simulink model "rtwdemo_slcustcode"  (Simulink 7.6)
settings: Solver=FixedStepDiscrete  StartTime=0.0  StopTime=48  FixedStep=1  RelTol=1e-3
libraries: rtwdemowidgets x3
Description:
  | Integrating Legacy Code Using Custom Code Blocks
settings Model: Creator=The MathWorks Inc.  ParamWorkspaceSource=ReferencedWorkspace  CovMetricSettings=d  ExtModeTrigMode=oneshot  ExtModeArmWhenConnect=off  ExtModeAutoUpdateStatusClock=off
settings MATStruct: SampleTime=1  Offset=0  Priority=[20.0]
settings DataIOCC: LimitDataPoints=off  SaveFormat=StructureWithTime  SaveOutput=off  SaveTime=off  SignalLoggingName=sigsOut
settings OptimizationCC: InlineParams=on  InlineInvariantSignals=on  StateBitsets=on  DataBitsets=on  UseTempVars=on  EfficientFloat2IntCast=on  EfficientMapNaN2IntZero=off
settings DebuggingCC: CheckExecutionContextPreStartOutputMsg=on  CheckExecutionContextRuntimeOutputMsg=on  SolverPrmCheckMsg=none  IntegerOverflowMsg=none  StrictBusMsg=ErrorOnBusTreatedAsVector
settings HardwareCC: ProdIntDivRoundTo=Zero  ProdEndianess=LittleEndian  ProdHWDeviceType=Generic->32-bit Embedded Processor  TargetHWDeviceType=Generic->32-bit Embedded Processor
settings ModelReferenceCC: UpdateModelReferenceTargets=IfOutOfDate
settings RTWCC: TLCOptions=-p0 -aWarnNonSaturatedBlocks=0  GenerateReport=on  RTWVerbose=off  ProcessScript=grt_make_rtw_hook  LaunchReport=on
settings RTWCC: CustomSourceCode=|
  | /* Declared from Configration Parameters RTW Custom Code Page (Source file) */
  | int_T GLOBAL_INT2 = -1;
settings RTWCC: CustomInitializer=|
  | /* Declared from Configuration Parameters RTW Custom Code Page (Initialize function) */
  | GLOBAL_INT2 = 1;
settings CodeAppCC: ForceParamTrailComments=on
settings GRTTargetCC: TargetFcnLib=ansi_tfl_tmw.mat

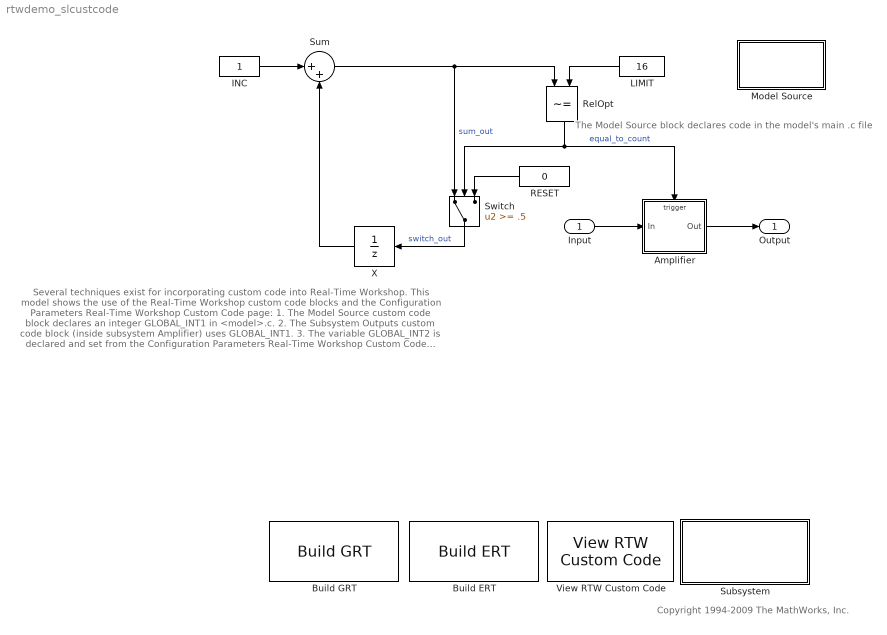
== system rtwdemo_slcustcode ==
  note: Several techniques exist for incorporating custom code into Real-Time Workshop.  This model
      | shows the use of the Real-Time Workshop custom code blocks and the Configuration Parameters
      | Real-Time Workshop Custom Code page:
      |
      | 1. The Model Source custom code block declares an integer GLOBAL_INT1 in <model>.c.
      | 2. The Subsystem Outputs custom code block (inside subsystem Amplifier) uses GLOBAL_INT1.
      | 3. The variable GLOBAL_INT2 is declared and set from the Configuration Parameters Real-Time
      |     Workshop Custom Code page, from the "Source file" and "Initialize function," respectively.
      |
      | Some overlap exists between custom code blocks and custom code specified using configuration
      | parameters, but custom code blocks provide much finer granularity of code placement, and have
      | the advantage of being graphical.
  note: The Model Source block
      | declares code in the
      | model's main .c file
  note: Copyright 1994-2009 The MathWorks, Inc.
  Input : Inport  OutDataTypeStr=int32  PortDimensions=1  SampleTime=1
  Amplifier : Subsystem  TreatAsAtomicUnit=on
  Build ERT : rtwdemowidgets/Build ERT  SystemSampleTime=-1  attrib_overrides={'IncludeMdlTerminateFcn'}
  Build GRT : rtwdemowidgets/Build GRT  SystemSampleTime=-1  attrib_overrides={}
  INC : Constant
  LIMIT : Constant  Value=16
  Model Source : Subsystem
      settings: CopyFcn=cccopyfcn(gcb)  OpenFcn=ccopenfcn('Model Source')
      mask Type: Model Source
      mask Description: Add code to the model .c file
      mask Help: This source file block contains text fields to insert custom user code at the top and bottom of model.c file.
      mask Display: disp('Model\nSource');
  RESET : Constant  Value=0
  RelOpt : RelationalOperator  Operator=~=  InputSameDT=on
  Subsystem : Subsystem
      settings: OpenFcn=custcode
      mask Display:
      | disp(['View Custom\nCode ',...
      | 	  'Library\n(double-click)'])
  Sum : Sum  Inputs=|++  InputSameDT=on  OutDataTypeStr=Inherit: Same as first input
  Switch : Switch  Threshold=.5  SaturateOnIntegerOverflow=on  InputSameDT=on
  View RTW Custom Code : rtwdemowidgets/View RTW Custom Code  SystemSampleTime=-1
  X : UnitDelay  StateIdentifier=X
  Output : Outport
  wires:
  INC/1 -> Sum/1
  X/1 -> Sum/2
  Switch/1 -> X/1  "switch_out"
  Sum/1 -> Switch/1, RelOpt/1  "sum_out"
  LIMIT/1 -> RelOpt/2
  Input/1 -> Amplifier/1(In)
  RESET/1 -> Switch/3
  RelOpt/1 -> Switch/2, Amplifier/Trigger  "equal_to_count"
  Amplifier/1(Out) -> Output/1

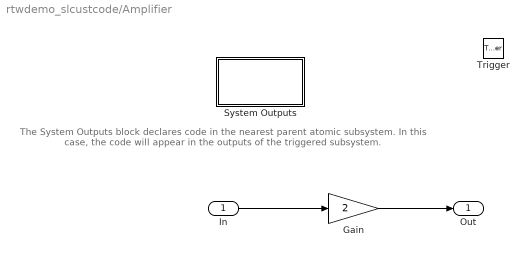
== system rtwdemo_slcustcode/Amplifier ==
  note: The System Outputs block declares code in the nearest
      | parent atomic subsystem.  In this case, the code will
      | appear in the outputs of the triggered subsystem.
  In : Inport
  Trigger : TriggerPort
  Gain : Gain  Gain=2  OutDataTypeStr=Inherit: Same as input  ParamDataTypeStr=Inherit: Same as input
  System Outputs : Subsystem
      settings: CopyFcn=cccopyfcn(gcb)  OpenFcn=ccopenfcn('System Outputs Function')
      mask Type: System Outputs
      mask Description: Add code to a systems Outputs function
      mask Help: This block contains text fields to insert custom user code sections at the declaration, execution and exit sections of the systems outputs function.  By placing this block inside a subsystem, the custom user code will appear in that subsystems function.
      mask Display: disp('System\nOutputs');
  Out : Outport  InitialOutput=0
  wires:
  In/1 -> Gain/1
  Gain/1 -> Out/1

== system rtwdemo_slcustcode/Model Source ==

== system rtwdemo_slcustcode/Subsystem ==

== system rtwdemo_slcustcode/Amplifier/System Outputs ==
